simulink model "ForwardVehicleSensorFusionTestBench"  (R2022a)
settings: Solver=FixedStepAuto  StartTime=0.0  StopTime=scenario.StopTime  RelTol=1e-3
PostLoadFcn:
  | helperSLForwardVehicleSensorFusionSetup
values from neighbouring files (symbols this model uses):
  camera = cameraParams(egoVehicle)    [helperSLForwardVehicleSensorFusionSetup.m]
  vehSim3D = repmat(     struct(         'Length', 0,         'RearOverhang', 0,         'InitialPos',[0 0 0],         'InitialRot',[0 0 0]),     numVehicles,1)    [helperSLForwardVehicleSensorFusionSetup.m]
undefined symbols (not defined in the file or in its folder): Ts
libraries: drivingscenarioandsensors x8, sim3dautolib x6, sim3dprobsensorlib x1, sim3dlib x1, drivingsim3d x1
CloseFcn:
  | helperSLForwardVehicleSensorFusionCleanUp
settings Model: SILPILSystemUnderTest=refmodels  Creator=The MathWorks, Inc.  LastModifiedBy=The MathWorks, Inc.
settings SolverCC: AlgebraicLoopSolver=TrustRegion  MaxZcPerStep=1
settings DataIOCC: SaveOutput=off  SaveTime=off  ReturnWorkspaceOutputs=off
settings OptimizationCC: ZeroExternalMemoryAtStartup=off  ZeroInternalMemoryAtStartup=off
settings DebuggingCC: ParameterPrecisionLossMsg=none  UnconnectedInputMsg=warning  UnconnectedOutputMsg=warning  UnconnectedLineMsg=warning  PregeneratedLibrarySubsystemCodeDiagnostic=none  SFMachineParentedDataDiag=warning  ArithmeticOperatorsInVariantConditions=warning
settings HardwareCC: ProdLongLongMode=on
settings SFSimCC: SimUseLocalCustomCode=off  SimTargetLang=C++
settings RTWCC: RTWUseLocalCustomCode=off  TargetLang=C++  DLArmComputeVersion=19.05
settings GRTTargetCC: TargetLangStandard=C++03 (ISO)  CodeInterfacePackaging=C++ class  RTWCAPISignals=on
settings ConfigComp: CovScope=ReferencedModels  CovIncludeTopModel=off

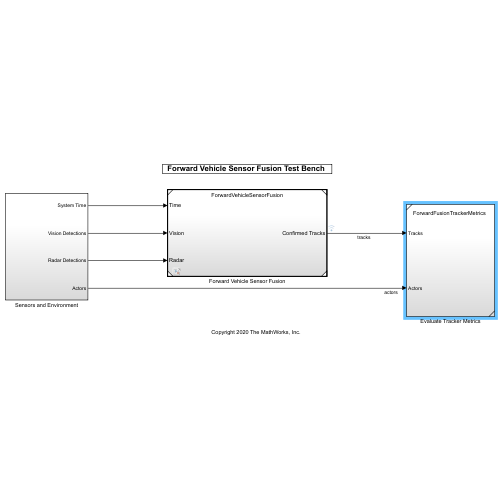
[thumbnail: Simulink's stored preview of the top-level diagram]
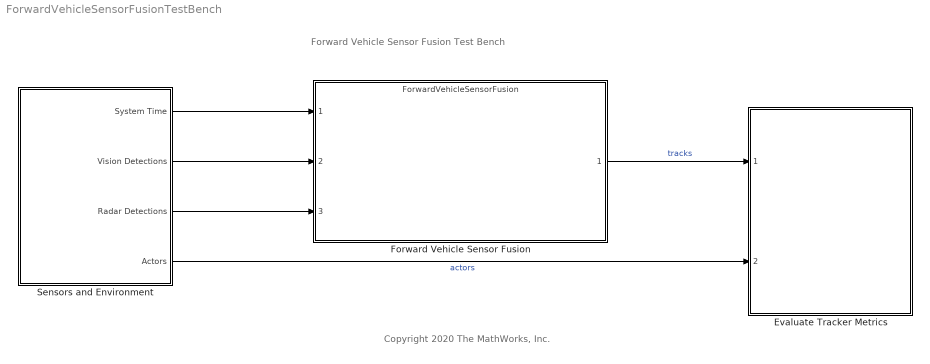
== system ForwardVehicleSensorFusionTestBench ==
  note: Forward Vehicle Sensor Fusion Test Bench
  note: Copyright 2020 The MathWorks, Inc.
  Evaluate Tracker Metrics : Subsystem  ReferencedSubsystem=ForwardFusionTrackerMetrics
  Forward Vehicle Sensor Fusion : ModelReference  ModelNameDialog=ForwardVehicleSensorFusion.slx  SimulationMode=Normal  CodeInterface=Top model  ModelReferenceVersion=5.7
  Sensors and Environment : Subsystem  VariantControl=1
  wires:
  Sensors and Environment/1(System Time) -> Forward Vehicle Sensor Fusion/1
  Sensors and Environment/3(Radar Detections) -> Forward Vehicle Sensor Fusion/3
  Sensors and Environment/4(Actors) -> Evaluate Tracker Metrics/2  "actors"
  Forward Vehicle Sensor Fusion/1 -> Evaluate Tracker Metrics/1  "tracks"
  Sensors and Environment/2(Vision Detections) -> Forward Vehicle Sensor Fusion/2

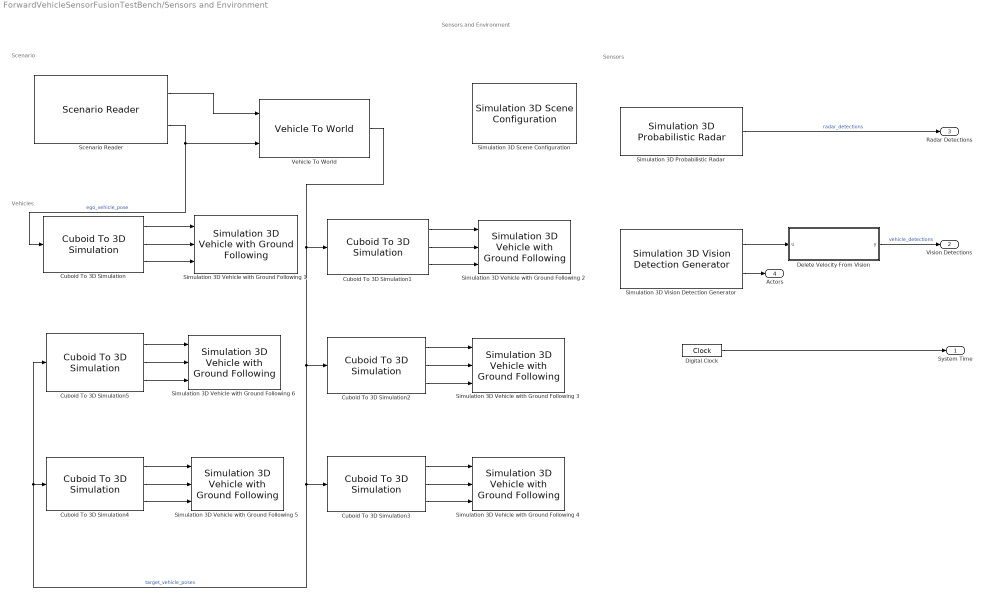
== system ForwardVehicleSensorFusionTestBench/Sensors and Environment ==
  note: Sensors
  note: Sensors and Environment
  note: Scenario
  note: Vehicles
  Cuboid To 3D Simulation : drivingscenarioandsensors/Cuboid To 3D Simulation  SpecifyActorID=off  ActorIDToConvert=1  SimulateUsing=Interpreted execution
      settings: SourceProductBaseCode=DR
  Cuboid To 3D Simulation1 : drivingscenarioandsensors/Cuboid To 3D Simulation  SpecifyActorID=on  ActorIDToConvert=2  SimulateUsing=Interpreted execution
      settings: SourceProductBaseCode=DR
  Cuboid To 3D Simulation2 : drivingscenarioandsensors/Cuboid To 3D Simulation  SpecifyActorID=on  ActorIDToConvert=3  SimulateUsing=Interpreted execution
      settings: SourceProductBaseCode=DR
  Cuboid To 3D Simulation3 : drivingscenarioandsensors/Cuboid To 3D Simulation  SpecifyActorID=on  ActorIDToConvert=4  SimulateUsing=Interpreted execution
      settings: SourceProductBaseCode=DR
  Cuboid To 3D Simulation4 : drivingscenarioandsensors/Cuboid To 3D Simulation  SpecifyActorID=on  ActorIDToConvert=5  SimulateUsing=Interpreted execution
      settings: SourceProductBaseCode=DR
  Cuboid To 3D Simulation5 : drivingscenarioandsensors/Cuboid To 3D Simulation  SpecifyActorID=on  ActorIDToConvert=6  SimulateUsing=Interpreted execution
      settings: SourceProductBaseCode=DR
  "Delete Velocity From Vision " : MATLAB Function  TreatAsAtomicUnit=on  mask(Pack vision detections){structInit=Simulink.Bus.createMATLABStruct('BusVision'), measurementNoise=camera.MeasurementNoise}
      mask prompts: structInit "Output struct"; measurementNoise "Measurement noise"
      mask help: Packs vision detections to match bus used by vision processing algorithm. This includes replacing the measurement noise and disabling the velocity measurement.
  Digital Clock : DigitalClock  SampleTime=Ts
  Scenario Reader : drivingscenarioandsensors/Scenario Reader  ScenarioSource=From workspace  ScenarioFileName=dblLaneChangeDrivingScenario.mat  ScenarioVariableName=scenario  OutputCoordinateSystem=Vehicle coordinates  EgoVehicleSource=Scenario  EgoVehicleActorID=1  OrientVehiclesOnRoad=off  OutputEgoVehiclePose=on  OutputEgoVehicleState=off  SampleTime=0.1  LaneBoundaryOutput=None  LaneBoundaryDistance=0:0.5:70  LaneBoundaryLocation=Center of lane markings  BusNameSource=Auto  BusName=BusActors  BusNumActorsSource=Scenario  BusNumActors=100  BusName2Source=Auto  BusName2=BusLaneBoundaries  BusNumLaneBoundariesSource=Scenario  BusNumLaneBoundaries=10  BusName3Source=Auto  BusName3=BusEgoActor  BusName4Source=Auto  BusName4=BusEgoState  ShowCoordinateLabels=on  SimulateUsing=Interpreted execution
  Simulation 3D Probabilistic Radar : sim3dprobsensorlib/Simulation 3D Probabilistic Radar  Priority=1  sensorTag=Sim3dSensor2  sensorId=2  sensorName=Sim3dSensor2  vehTagList={'Scene Origin';'SimulinkVehicle1';'SimulinkVehicle2';'SimulinkVehicle3';'SimulinkVehicle4';'SimulinkVehicle5';'SimulinkVehicle6'}  vehTag=SimulinkVehicle1  mountLoc=Origin  offsetFlag=on  tmountOffset=radar.PositionSim3d  rmountOffset=radar.Rotation  AzimuthResolution=0.8  ElevationResolution=8  RangeResolution=1  RangeRateResolution=1  AzimuthBiasFraction=0.1  ElevationBiasFraction=0.1  RangeBiasFraction=0.05  RangeRateBiasFraction=0.05  FieldOfView=radar.FieldOfView  DetectionRange=radar.DetectionRanges  RangeRateLimits=[ -100, 100 ]  DetectionProbability=0.9  FalseAlarmRate=1e-6  ReferenceRange=100  ReferenceRCS=0  HasElevation=off  HasRangeRate=on  HasNoise=off  HasFalseAlarms=off  InitialSeedSource=Repeatable  InitialSeed=0  MaxNumDetections=50  DetectionCoordinates=Sensor spherical  SpecifyOutputBusName=off  BusName=BusSimulation3DRadarTruthSensor  SampleTime=-1  mountPoint=[2.424 0 0.8]  mountOrientation=[0 0 0]  aMode=3  ID=2
      settings: SourceProductBaseCode=VE,AE,DR,UV,VE
      settings: AttributesFormatString=|
      | -------------------------------------
      | FieldOfView = %<FieldOfView>
      | AzimuthResolution = %<AzimuthResolution>
      | DetectionCoordinates = %<DetectionCoordinates>
      | mountLoc = %<mountLoc>
      | tmountOffset = %<tmountOffset>
      | rmountOffset = %<rmountOffset>
      | Priority = %<Priority>
  Simulation 3D Scene Configuration : sim3dlib/Simulation 3D Scene Configuration  Priority=0  ProjectFormat=Default Scenes  SceneDesc=Curved road  ProjectName=/mathworks/devel/bat/BR2022ad/build/matlab/toolbox/shared/sim3d_projects/automotive_project/UE4/LinuxNoEditor/AutoVrtlEnv.sh  ScenePath=/Game/Maps/HwStrght  vehTagList={'Scene Origin';'SimulinkVehicle1';'SimulinkVehicle2';'SimulinkVehicle3';'SimulinkVehicle4';'SimulinkVehicle5';'SimulinkVehicle6'}  vehTag=SimulinkVehicle1  OpVisEn=off  Ts=0.1  EnableWindow=on  EnableRemoteAccess=off  EnableWeather=off  SunAltitude=40.0  SunAzimuth=90  clouds=10  wind=1  fog=0  rain=0  sensorTag=MainCamera1  sensorId=1  sensorName=MainCamera1  mountLoc=Origin  offsetFlag=off  tmountOffset=[0, 0, 0]  rmountOffset=[0, 0, 0]  HorizontalResolution=1280  VerticalResolution=720  HorizontalFOV=60  mountPoint=[0 0 0]  mountOrientation=[0 0 0]  aMode=3  ID=1
      settings: SourceProductBaseCode=VE,AE,DR,UV,VE
      settings: AttributesFormatString=|
      | -------------------------------------
      | SceneName = %<SceneDesc>
      | Priority = %<Priority>
  Simulation 3D Vehicle with Ground Following 1 : sim3dautolib/Simulation 3D Vehicle with Ground Following  Priority=-1  PassVehMesh=Sedan  MeshPath=/MathWorksSimulation/Vehicles/Muscle/Meshes/SK_MuscleCar.SK_MuscleCar  TrackWidth=1.9  WheelBase=3  WheelRadius=0.35  VehColor=Blue  InitialPos=vehSim3D(1).InitialPos  InitialRot=vehSim3D(1).InitialRot  ActorName=SimulinkVehicle1  SampleTime=-1  ActorType=SimulinkVehicle  ID=1  aMode=3  ActorTag=SimulinkVehicle1  CoordinateScheme=ISO  VehLightsControl=off  HeadlightColor=[ 1, 1, 1 ]  HighBeamIntensity=100000  LowBeamIntensity=60000  HighBeamConeAngle=70  LowBeamConeAngle=70  LeftHeadlightOrientation=[ 0, 0 ]  RightHeadlightOrientation=[ 0, 0 ]  BrakelightIntensity=500  ReverselightIntensity=500  SignallightIntensity=500  SignallightPeriod=1  SignalPulseWidth=50  TransformOutportEnabled=off
      settings: SourceProductBaseCode=VE,AE,DR,UV,VE
      settings: AttributesFormatString=|
      | --------------------------------------
      | ActorName = %<ActorName>
      | PassVehMesh = %<PassVehMesh>
      | VehColor = %<VehColor>
      | InitialPos = %<InitialPos>
      | InitialRot = %<InitialRot>
      | Priority = %<Priority>
  Simulation 3D Vehicle with Ground Following 2 : sim3dautolib/Simulation 3D Vehicle with Ground Following  Priority=-1  PassVehMesh=Sedan  MeshPath=/MathWorksSimulation/Vehicles/Muscle/Meshes/SK_MuscleCar.SK_MuscleCar  TrackWidth=1.9  WheelBase=3  WheelRadius=0.35  VehColor=Red  InitialPos=vehSim3D(2).InitialPos  InitialRot=vehSim3D(2).InitialRot  ActorName=SimulinkVehicle2  SampleTime=-1  ActorType=SimulinkVehicle  ID=2  aMode=3  ActorTag=SimulinkVehicle2  CoordinateScheme=ISO  VehLightsControl=off  HeadlightColor=[ 1, 1, 1 ]  HighBeamIntensity=100000  LowBeamIntensity=60000  HighBeamConeAngle=70  LowBeamConeAngle=70  LeftHeadlightOrientation=[ 0, 0 ]  RightHeadlightOrientation=[ 0, 0 ]  BrakelightIntensity=500  ReverselightIntensity=500  SignallightIntensity=500  SignallightPeriod=1  SignalPulseWidth=50  TransformOutportEnabled=off
      settings: SourceProductBaseCode=VE,AE,DR,UV,VE
      settings: AttributesFormatString=|
      | --------------------------------------
      | ActorName = %<ActorName>
      | PassVehMesh = %<PassVehMesh>
      | VehColor = %<VehColor>
      | InitialPos = %<InitialPos>
      | InitialRot = %<InitialRot>
      | Priority = %<Priority>
  Simulation 3D Vehicle with Ground Following 3 : sim3dautolib/Simulation 3D Vehicle with Ground Following  Priority=-1  PassVehMesh=Muscle car  MeshPath=/MathWorksSimulation/Vehicles/Muscle/Meshes/SK_MuscleCar.SK_MuscleCar  TrackWidth=1.9  WheelBase=3  WheelRadius=0.35  VehColor=Black  InitialPos=vehSim3D(3).InitialPos  InitialRot=vehSim3D(3).InitialRot  ActorName=SimulinkVehicle3  SampleTime=-1  ActorType=SimulinkVehicle  ID=3  aMode=3  ActorTag=SimulinkVehicle3  CoordinateScheme=ISO  VehLightsControl=off  HeadlightColor=[ 1, 1, 1 ]  HighBeamIntensity=100000  LowBeamIntensity=60000  HighBeamConeAngle=70  LowBeamConeAngle=70  LeftHeadlightOrientation=[ 0, 0 ]  RightHeadlightOrientation=[ 0, 0 ]  BrakelightIntensity=500  ReverselightIntensity=500  SignallightIntensity=500  SignallightPeriod=1  SignalPulseWidth=50  TransformOutportEnabled=off
      settings: SourceProductBaseCode=VE,AE,DR,UV,VE
      settings: AttributesFormatString=|
      | --------------------------------------
      | ActorName = %<ActorName>
      | PassVehMesh = %<PassVehMesh>
      | VehColor = %<VehColor>
      | InitialPos = %<InitialPos>
      | InitialRot = %<InitialRot>
      | Priority = %<Priority>
  Simulation 3D Vehicle with Ground Following 4 : sim3dautolib/Simulation 3D Vehicle with Ground Following  Priority=-1  PassVehMesh=Hatchback  MeshPath=/MathWorksSimulation/Vehicles/Muscle/Meshes/SK_MuscleCar.SK_MuscleCar  TrackWidth=1.9  WheelBase=3  WheelRadius=0.35  VehColor=Orange  InitialPos=vehSim3D(4).InitialPos  InitialRot=vehSim3D(4).InitialRot  ActorName=SimulinkVehicle4  SampleTime=-1  ActorType=SimulinkVehicle  ID=4  aMode=3  ActorTag=SimulinkVehicle4  CoordinateScheme=ISO  VehLightsControl=off  HeadlightColor=[ 1, 1, 1 ]  HighBeamIntensity=100000  LowBeamIntensity=60000  HighBeamConeAngle=70  LowBeamConeAngle=70  LeftHeadlightOrientation=[ 0, 0 ]  RightHeadlightOrientation=[ 0, 0 ]  BrakelightIntensity=500  ReverselightIntensity=500  SignallightIntensity=500  SignallightPeriod=1  SignalPulseWidth=50  TransformOutportEnabled=off
      settings: SourceProductBaseCode=VE,AE,DR,UV,VE
      settings: AttributesFormatString=|
      | --------------------------------------
      | ActorName = %<ActorName>
      | PassVehMesh = %<PassVehMesh>
      | VehColor = %<VehColor>
      | InitialPos = %<InitialPos>
      | InitialRot = %<InitialRot>
      | Priority = %<Priority>
  Simulation 3D Vehicle with Ground Following 5 : sim3dautolib/Simulation 3D Vehicle with Ground Following  Priority=-1  PassVehMesh=Small pickup truck  MeshPath=/MathWorksSimulation/Vehicles/Muscle/Meshes/SK_MuscleCar.SK_MuscleCar  TrackWidth=1.9  WheelBase=3  WheelRadius=0.35  VehColor=Green  InitialPos=vehSim3D(5).InitialPos  InitialRot=vehSim3D(5).InitialRot  ActorName=SimulinkVehicle5  SampleTime=-1  ActorType=SimulinkVehicle  ID=5  aMode=3  ActorTag=SimulinkVehicle5  CoordinateScheme=ISO  VehLightsControl=off  HeadlightColor=[ 1, 1, 1 ]  HighBeamIntensity=100000  LowBeamIntensity=60000  HighBeamConeAngle=70  LowBeamConeAngle=70  LeftHeadlightOrientation=[ 0, 0 ]  RightHeadlightOrientation=[ 0, 0 ]  BrakelightIntensity=500  ReverselightIntensity=500  SignallightIntensity=500  SignallightPeriod=1  SignalPulseWidth=50  TransformOutportEnabled=off
      settings: SourceProductBaseCode=VE,AE,DR,UV,VE
      settings: AttributesFormatString=|
      | --------------------------------------
      | ActorName = %<ActorName>
      | PassVehMesh = %<PassVehMesh>
      | VehColor = %<VehColor>
      | InitialPos = %<InitialPos>
      | InitialRot = %<InitialRot>
      | Priority = %<Priority>
  Simulation 3D Vehicle with Ground Following 6 : sim3dautolib/Simulation 3D Vehicle with Ground Following  Priority=-1  PassVehMesh=Sport utility vehicle  MeshPath=/MathWorksSimulation/Vehicles/Muscle/Meshes/SK_MuscleCar.SK_MuscleCar  TrackWidth=1.9  WheelBase=3  WheelRadius=0.35  VehColor=Blue  InitialPos=vehSim3D(6).InitialPos  InitialRot=vehSim3D(6).InitialRot  ActorName=SimulinkVehicle6  SampleTime=-1  ActorType=SimulinkVehicle  ID=6  aMode=3  ActorTag=SimulinkVehicle6  CoordinateScheme=ISO  VehLightsControl=off  HeadlightColor=[ 1, 1, 1 ]  HighBeamIntensity=100000  LowBeamIntensity=60000  HighBeamConeAngle=70  LowBeamConeAngle=70  LeftHeadlightOrientation=[ 0, 0 ]  RightHeadlightOrientation=[ 0, 0 ]  BrakelightIntensity=500  ReverselightIntensity=500  SignallightIntensity=500  SignallightPeriod=1  SignalPulseWidth=50  TransformOutportEnabled=off
      settings: SourceProductBaseCode=VE,AE,DR,UV,VE
      settings: AttributesFormatString=|
      | --------------------------------------
      | ActorName = %<ActorName>
      | PassVehMesh = %<PassVehMesh>
      | VehColor = %<VehColor>
      | InitialPos = %<InitialPos>
      | InitialRot = %<InitialRot>
      | Priority = %<Priority>
  Simulation 3D Vision Detection Generator : drivingsim3d/Simulation 3D Vision Detection Generator  Priority=1  sensorTag=Sim3dSensor255  sensorId=1  sensorName=Sim3dSensor1  vehTagList={'Scene Origin';'SimulinkVehicle1';'SimulinkVehicle2';'SimulinkVehicle3';'SimulinkVehicle4';'SimulinkVehicle5';'SimulinkVehicle6'}  vehTag=SimulinkVehicle1  mountLoc=Origin  offsetFlag=on  tmountOffset=camera.PositionSim3d  rmountOffset=camera.Rotation  DetectorOutput=Objects only  MaxNumDetections=20  MaxNumLanes=30  laneSampleDistances=0:0.5:9.5  BusNameSource=Property  BusName=BusObjectDetections  BusName2Source=Auto  BusName2=BusLaneDetections  MaxRange=camera.DetectionRanges(2)  BoundingBoxAccuracy=5  ProcessNoiseIntensity=5  MaxSpeed=50  MaxAllowedOcclusion=0.5  MinObjectImageSize=camera.MinObjectImageSize  DetectionProbability=0.9  FalsePositivesPerImage=0  MinLaneImageSize=[ 20, 3 ]  LaneBoundaryAccuracy=3  HasNoise=off  InitialSeedSource=Repeatable  InitialSeed=1  uniqueActorIdentifier=[]  actorClassInteger=0  cuboidLength=4.7  cuboidWidth=1.8  cuboidHeight=1.4  rotationalCenter={[-1.35, 0, 0]}  focalLength=camera.FocalLength  opticalCenter=camera.PrincipalPoint  imageSize=camera.ImageSize  radialDistortionCoefficients=[0, 0]  tangentialDistortionCoefficients=[0, 0]  cameraAxisSkew=0  actorTruthOutportEnabled=on  laneTruthOutportEnabled=off  SampleTime=-1  checkedSampleTime=0.1  mountPoint=[0.57 0 1.2]  mountOrientation=[0 0 0]  aMode=3  ID=1
      settings: SourceProductBaseCode=DR
  Vehicle To World : drivingscenarioandsensors/Vehicle To World  BusNameSource=Auto  BusName=BusVehicleToWorldActors  SimulateUsing=Interpreted execution
      settings: SourceProductBaseCode=DR
  System Time : Outport  VectorParamsAs1DForOutWhenUnconnected=off
  Vision Detections : Outport  Port=2  OutDataTypeStr=Bus:BusVision
  Radar Detections : Outport  Port=3
  Actors : Outport  Port=4
  wires:
  Cuboid To 3D Simulation/1 -> Simulation 3D Vehicle with Ground Following 1/1
  Cuboid To 3D Simulation/3 -> Simulation 3D Vehicle with Ground Following 1/3
  Cuboid To 3D Simulation/2 -> Simulation 3D Vehicle with Ground Following 1/2
  Cuboid To 3D Simulation1/2 -> Simulation 3D Vehicle with Ground Following 2/2
  Cuboid To 3D Simulation1/3 -> Simulation 3D Vehicle with Ground Following 2/3
  Cuboid To 3D Simulation1/1 -> Simulation 3D Vehicle with Ground Following 2/1
  Scenario Reader/1 -> Vehicle To World/1
  Scenario Reader/2 -> Cuboid To 3D Simulation/1, Vehicle To World/2  "ego_vehicle_pose"
  Simulation 3D Probabilistic Radar/1 -> Radar Detections/1  "radar_detections"
  Vehicle To World/1 -> Cuboid To 3D Simulation1/1, Cuboid To 3D Simulation2/1, Cuboid To 3D Simulation3/1, Cuboid To 3D Simulation5/1, Cuboid To 3D Simulation4/1  "target_vehicle_poses"
  Cuboid To 3D Simulation2/2 -> Simulation 3D Vehicle with Ground Following 3/2
  Cuboid To 3D Simulation2/1 -> Simulation 3D Vehicle with Ground Following 3/1
  Cuboid To 3D Simulation2/3 -> Simulation 3D Vehicle with Ground Following 3/3
  Cuboid To 3D Simulation3/2 -> Simulation 3D Vehicle with Ground Following 4/2
  Cuboid To 3D Simulation3/1 -> Simulation 3D Vehicle with Ground Following 4/1
  Cuboid To 3D Simulation3/3 -> Simulation 3D Vehicle with Ground Following 4/3
  Cuboid To 3D Simulation4/2 -> Simulation 3D Vehicle with Ground Following 5/2
  Cuboid To 3D Simulation4/1 -> Simulation 3D Vehicle with Ground Following 5/1
  Cuboid To 3D Simulation4/3 -> Simulation 3D Vehicle with Ground Following 5/3
  Cuboid To 3D Simulation5/2 -> Simulation 3D Vehicle with Ground Following 6/2
  Cuboid To 3D Simulation5/1 -> Simulation 3D Vehicle with Ground Following 6/1
  Cuboid To 3D Simulation5/3 -> Simulation 3D Vehicle with Ground Following 6/3
  Digital Clock/1 -> System Time/1
  Simulation 3D Vision Detection Generator/1 -> "Delete Velocity From Vision "/1(u)
  "Delete Velocity From Vision "/1(y) -> Vision Detections/1  "vehicle_detections"
  Simulation 3D Vision Detection Generator/2 -> Actors/1

== matlab function ForwardVehicleSensorFusionTestBench/Sensors and Environment/Delete Velocity From Vision  ==
  data: u input; y output Bus: BusVision; structInit parameter; measurementNoise parameter
function y = deleteVelocityFromVision(u,structInit,measurementNoise)

y = structInit;
y.NumDetections = u.NumDetections;
y.IsValidTime = u.IsValidTime;
for n = 1:u.NumDetections
    y.Detections(n).Time = u.Detections(n).Time;
    y.Detections(n).Measurement = u.Detections(n).Measurement(1:3);
    y.Detections(n).MeasurementNoise = measurementNoise;
    y.Detections(n).SensorIndex = u.Detections(n).SensorIndex;
    y.Detections(n).ObjectClassID = u.Detections(n).ObjectClassID;
    y.Detections(n).ObjectAttributes = u.Detections(n).ObjectAttributes;
    y.Detections(n).MeasurementParameters = u.Detections(n).MeasurementParameters;
    y.Detections(n).MeasurementParameters.HasVelocity = false;
end
